simulink model "statespace"  (R2017a)
settings: Solver=VariableStepAuto  StartTime=0.0  StopTime=10.0  RelTol=1e-3
values from neighbouring files (symbols this model uses):
  theta_til = theta_ref - theta    [trajectory_following.m]
  v = 0.5    [24_abril_sesh.mat]    (also in 26_abril_sesh.mat = 2; Gain_tune.m; Simulation.m = timeseries(vt); TestSimulink.m = timeseries(v_vec(i)))
undefined symbols (not defined in the file or in its folder): w_atual
settings Model: Creator=joaogarcia  LastModifiedBy=joaogarcia

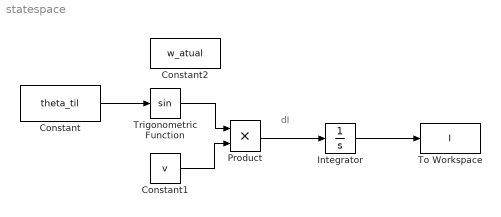
== system statespace ==
  note: dI
  Constant : Constant  Value=theta_til
  Constant1 : Constant  Value=v
  Constant2 : Constant  Value=w_atual
  Integrator : Integrator
  Product : Product
  To Workspace : ToWorkspace  VariableName=I  SaveFormat=Timeseries  SampleTime=-1
  Trigonometric Function : Trigonometry
  wires:
  Constant1/1 -> Product/2
  Constant/1 -> Trigonometric Function/1
  Trigonometric Function/1 -> Product/1
  Product/1 -> Integrator/1
  Integrator/1 -> To Workspace/1
